simulink model "visualisation"  (R2022b)
settings: Solver=VariableStepAuto  StartTime=0.0  StopTime=10.0  RelTol=1e-3
libraries: sim3dlib x1, sim3dautolib x1
settings Model: Creator=ok  LastModifiedBy=ok

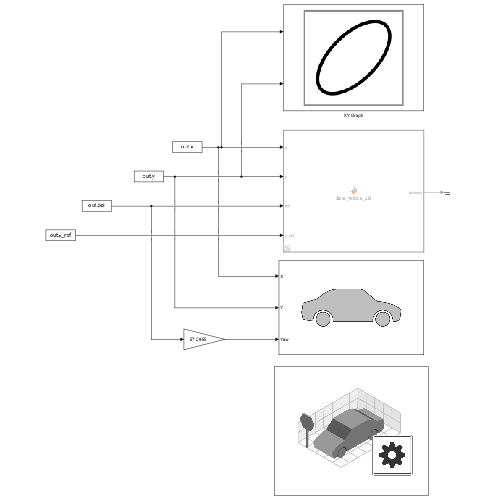
[thumbnail: Simulink's stored preview of the top-level diagram]
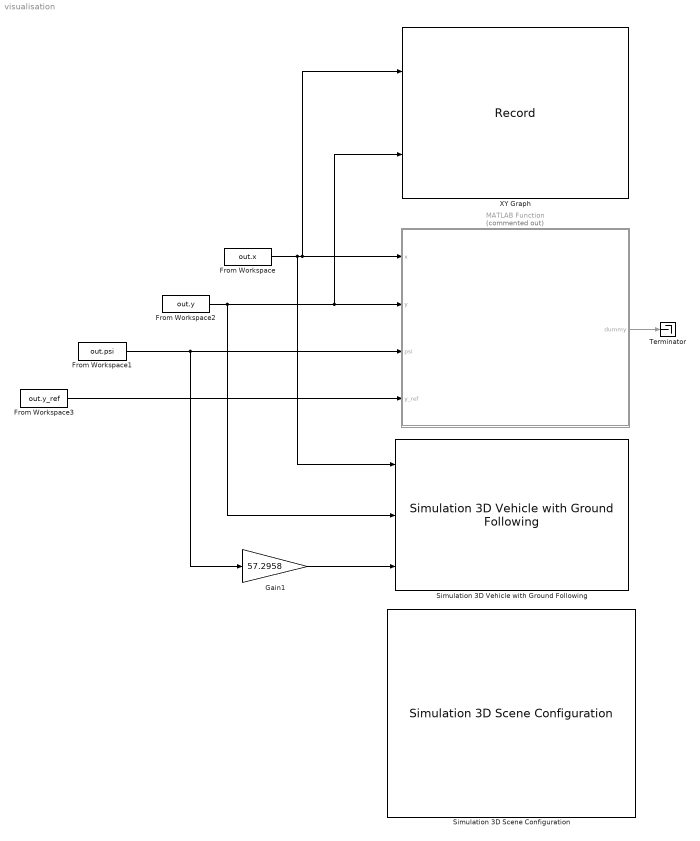
== system visualisation ==
  From Workspace : FromWorkspace  VariableName=out.x
  From Workspace1 : FromWorkspace  VariableName=out.psi
  From Workspace2 : FromWorkspace  VariableName=out.y
  From Workspace3 : FromWorkspace  VariableName=out.y_ref
  Gain1 : Gain  Gain=57.2958
  MATLAB Function : MATLAB Function  Commented=on  TreatAsAtomicUnit=on
  Simulation 3D Scene Configuration : sim3dlib/Simulation 3D Scene Configuration  Priority=0  ProjectFormat=Default Scenes  SceneDesc=Straight road  ProjectName=C:\Program Files\MATLAB\R2022b\toolbox\shared\sim3d_projects\automotive_project\UE4\WindowsNoEditor\VehicleSimulation.exe  ScenePath=/Game/Maps/HwStrght  EnableOpenDRIVE=off  vehTagList={'Scene Origin';'SimulinkVehicle1'}  vehTag=SimulinkVehicle1  OpVisEn=off  Ts=1/60  EnableWindow=on  EnableRemoteAccess=off  EnableWeather=off  SunAltitude=40.0  SunAzimuth=90  clouds=10  wind=1  fog=0  rain=0  EnableGeospatial=off  OriginHeight=200  OriginLatitude=40.744652  OriginLongitude=-73.988864  MapStyle=Aerial  AdditionalAssetIDs=[]  UseAdvancedSunSky=off  SolarTime=11  TimeZone=-5  Day=21  Month=9  Year=2022  UseDaylightSavingTime=on  DSTStartDay=10  DSTStartMonth=3  DSTEndDay=3  DSTEndMonth=11  DSTSwitchHour=2  sensorTag=MainCamera2  sensorId=2  sensorName=MainCamera2  mountLoc=Origin  offsetFlag=off  tmountOffset=[0, 0, 0]  rmountOffset=[0, 0, 0]  HorizontalResolution=1280  VerticalResolution=720  HorizontalFOV=60  mountPoint=[0 0 0]  mountOrientation=[0 0 0]  aMode=3  ID=2  GeoTrigger=Inactive
      settings: LibrarySourceBlock=drivingsim3d/Simulation 3D Scene Configuration
  Simulation 3D Vehicle with Ground Following : sim3dautolib/Simulation 3D Vehicle with Ground Following  Priority=-1  PassVehMesh=Small pickup truck  MeshPath=/MathWorksAutomotiveContent/Vehicles/Muscle/Meshes/SK_MuscleCar.SK_MuscleCar  TrackWidth=1.9  WheelBase=3  WheelRadius=0.35  VehColor=Orange  InitialPos=[0, 0, 0]  InitialRot=[0, 0, 90]  ActorName=SimulinkVehicle2  SampleTime=-1  ActorType=SimulinkVehicle  ID=2  aMode=3  ActorTag=SimulinkVehicle2  CoordinateScheme=ISO  VehLightsControl=off  HeadlightColor=[ 1, 1, 1 ]  HighBeamIntensity=100000  LowBeamIntensity=60000  HighBeamConeAngle=70  LowBeamConeAngle=70  LeftHeadlightOrientation=[ 0, 0 ]  RightHeadlightOrientation=[ 0, 0 ]  BrakelightIntensity=500  ReverselightIntensity=500  SignallightIntensity=500  SignallightPeriod=1  SignalPulseWidth=50  TransformOutportEnabled=off
      settings: LibrarySourceBlock=drivingsim3d/Simulation 3D Vehicle with Ground Following
  Terminator : Terminator
  XY Graph : Record  FileSettingsInternal="{\"entries\":[{\"content\":{\"excelSettings\":{\"content\":{},\"type\":\"Streamout.ExcelSettings\"}},\"type\":\"Streamout.FileSettingStorage\",\"uuid\":\"424a7271-1c28-4919-96f3-c3ddd62c1326\"}],\"packageUris\":[\"http://schema.mathworks.com/mf0/streamout_blocks/R2020a\"],\"version\":\"1.0\"}"  Layout=[1 1]  SignalsInternal="{\"entries\":[{\"content\":{\"signals\":[{\"content\":{\"blockPath\":[\"visualisation/XY Graph\"],\"channel\":[],\"dimensions\":[1],\"domain\":\"visualisation/XY Graph\",\"lineColor\":\"#7e2f8e\",\"plots\":[],\"port\":1,\"sid\":[\"\"],\"signalID\":922,\"signalName\":\"From\\nWorkspace\"},\"type\":\"RecordBlkView.Signal\",\"uuid\":\"baab0a3b-08eb-45eb-934d-8fd622ce3a02\"},{\"content\":{\"blockPath\":[\"visualisation/XY Graph\"],\"channel\":[],\"dimensions\":[1],\"domain\":\"visualisation/XY Graph\",\"lineColor\":\"#77ac30\",\"plots\":[],\"port\":2,\"sid\":[\"\"],\"signalID\":926,\"signalName\":\"From\\nWorkspace2\"},\"type\":\"RecordBlkView.Signal\",\"uuid\":\"04ebe1fa-14a5-45ff-9eae-455c0aaf322b\"}]},\"type\":\"RecordBlkView.InputSignals\",\"uuid\":\"8c9c14b2-cf3b-4012-a61d-7dc1a321b067\"}],\"packageUris\":[\"http://schema.mathworks.com/mf0/streamout_blocks/R2020a\"],\"version\":\"1.0\"}"  VisualizationBindings="{\"xyplotplugin\":{\"info\":[{\"series\":[],\"subplotID\":1}]}}"  CompatibilityTag=XY
  wires:
  MATLAB Function/1(dummy) -> Terminator/1
  From Workspace/1 -> Simulation 3D Vehicle with Ground Following/1, XY Graph/1, MATLAB Function/1(x)
  From Workspace2/1 -> Simulation 3D Vehicle with Ground Following/2, XY Graph/2, MATLAB Function/2(y)
  From Workspace1/1 -> Gain1/1, MATLAB Function/3(psi)
  From Workspace3/1 -> MATLAB Function/4(y_ref)
  Gain1/1 -> Simulation 3D Vehicle with Ground Following/3

== matlab function visualisation/MATLAB Function ==
  settings: updateMethod=DISCRETE
  data: x input; dummy output; y input; psi input; y_ref input
function dummy = draw_vehicle_2D(x, y, psi, y_ref)
%#codegen

coder.extrinsic('figure','clf','hold','grid','xlabel','ylabel', ...
                'title','legend','plot','fill','set','xlim','ylim', ...
                'drawnow','gca','gcf')

persistent hTraj hRef hCar Xveh Yveh Xref Yref isInit ax fig

dummy = 0;

if isempty(isInit)
    fig = figure(20);
    clf(fig);

    % Grande fenêtre
    set(fig,'Units','normalized');
    set(fig,'Position',[0.08 0.08 0.84 0.82]);

    ax = gca;
    hold(ax,'on');
    grid(ax,'on');

    % IMPORTANT : ne pas mettre axis equal
    set(ax,'Units','normalized');
    set(ax,'Position',[0.06 0.10 0.90 0.82]);

    xlabel(ax,'X [m]','FontSize',14);
    ylabel(ax,'Y [m]','FontSize',14);
    title(ax,'Suivi 2D du vehicule sur route','FontSize',16,'FontWeight','bold');

    % Rouge d'abord
    hTraj = plot(ax,0,0,'r-','LineWidth',2);

    % Bleu ensuite pour qu'il soit au-dessus
    hRef  = plot(ax,0,0,'b--o', ...
        'LineWidth',3, ...
        'MarkerSize',4, ...
        'MarkerFaceColor','b');

    % Rectangle véhicule
    hCar  = fill(ax,0,0,'r','EdgeColor','k','LineWidth',1.5);

    legend(ax, ...
        'Trajectoire reelle', ...
        'Route de reference', ...
        'Vehicule', ...
        'Location','northwest');

    Xveh = [];
    Yveh = [];
    Xref = [];
    Yref = [];

    isInit = true;
end

% Historique
Xveh = [Xveh, x];
Yveh = [Yveh, y];

Xref = [Xref, x];
Yref = [Yref, y_ref];

% Mise à jour courbes
set(hTraj,'XData',Xveh,'YData',Yveh);
set(hRef ,'XData',Xref,'YData',Yref);

% Rectangle du véhicule
L = 3.0;
W = 1.6;

corners = [ L/2,  W/2;
            L/2, -W/2;
           -L/2, -W/2;
           -L/2,  W/2]';

R = [cos(psi) -sin(psi);
     sin(psi)  cos(psi)];

rot = R * corners;

Xcar = rot(1,:) + x;
Ycar = rot(2,:) + y;

set(hCar,'XData',Xcar,'YData',Ycar);

% Axes qui remplissent bien la fenêtre
xmin = min([Xveh Xref]);
xmax = max([Xveh Xref]);

if isempty(xmin) || isempty(xmax)
    xmin = 0;
    xmax = 10;
end

if (xmax - xmin) < 40
    xc = 0.5*(xmin + xmax);
    xmin = xc - 20;
    xmax = xc + 20;
end

ymin = min([Yveh Yref]);
ymax = max([Yveh Yref]);

if isempty(ymin) || isempty(ymax)
    ymin = -5;
    ymax = 5;
end

if (ymax - ymin) < 12
    yc = 0.5*(ymin + ymax);
    ymin = yc - 6;
    ymax = yc + 6;
else
    ymin = ymin - 1;
    ymax = ymax + 1;
end

xlim(ax,[xmin xmax]);
ylim(ax,[ymin ymax]);

drawnow;
